simulink model "Milestone3_Code_JanasWork"  (R2023a)
settings: Solver=FixedStepDiscrete  StartTime=0.0  StopTime=100  FixedStep=0.01  RelTol=1e-3  EnableMultiTasking=on
undefined symbols (not defined in the file): DiscIntNeverNeededParam
libraries: arduinolib x14, simulink x3, hdlsllib x2, slpidlib x1, mobileRoboticsTrainingLib x1, arduinosensorlib x1
(part 1 of 2)
settings Model: NumberOfSteps=50  PacingRate=1000  ExtModeTrigDuration=2  Creator=Boitumelo  LastModifiedBy=27747
settings OptimizationCC: EnhancedBackFolding=on  PassReuseOutputArgsAs=Individual arguments  ZeroExternalMemoryAtStartup=off  ZeroInternalMemoryAtStartup=off  MaxStackSize=64  OptimizeBlockOrder=speed  DifferentSizesBufferReuse=on  OptimizationCustomize=off  EfficientTunableParamExpr=on
settings DebuggingCC: ParameterTunabilityLossMsg=error  UnconnectedInputMsg=warning  UnconnectedOutputMsg=warning  UnconnectedLineMsg=warning
settings HardwareCC: ProdBitPerPointer=32  ProdBitPerSizeT=32  ProdBitPerPtrDiffT=32  ProdLargestAtomicInteger=Long  ProdLargestAtomicFloat=Double  ProdWordSize=32  ProdHWDeviceType=ARM Compatible->ARM Cortex  UseEmbeddedCoderFeatures=off  UseSimulinkCoderFeatures=off
settings ModelReferenceCC: EnableRefExpFcnMdlSchedulingChecks=on
settings SFSimCC: MATLABDynamicMemAlloc=off
settings RTWCC: Description=Embedded Coder  SystemTargetFile=ert.tlc  HardwareBoard=Arduino Nano 33 IoT  TemplateMakefile=ert_default_tmf  Toolchain=Arduino ARM  BuildConfiguration=Faster Runs  DLArmComputeVersion=19.05
settings CodeAppCC: ForceParamTrailComments=on  IgnoreCustomStorageClasses=off  OperatorAnnotations=on  SimulinkDataObjDesc=on  SFDataObjDesc=on  InsertBlockDesc=on
settings ERTTargetCC: SupportContinuousTime=on  SupportNonInlinedSFcns=on  SupportVariableSizeSignals=on  ExtModeTransport=2  ExtModeStaticAlloc=on  ExtModeAutomaticAllocSize=off  ExtModeStaticAllocSize=8192  ExtModeMexFile=ext_xcp  ExtModeIntrfLevel=Level2 - Open

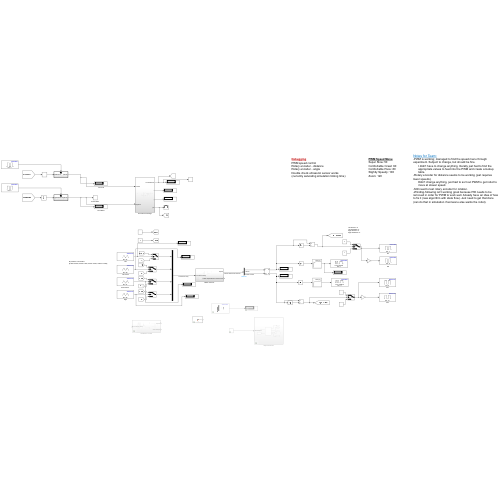
[thumbnail: Simulink's stored preview of the top-level diagram]
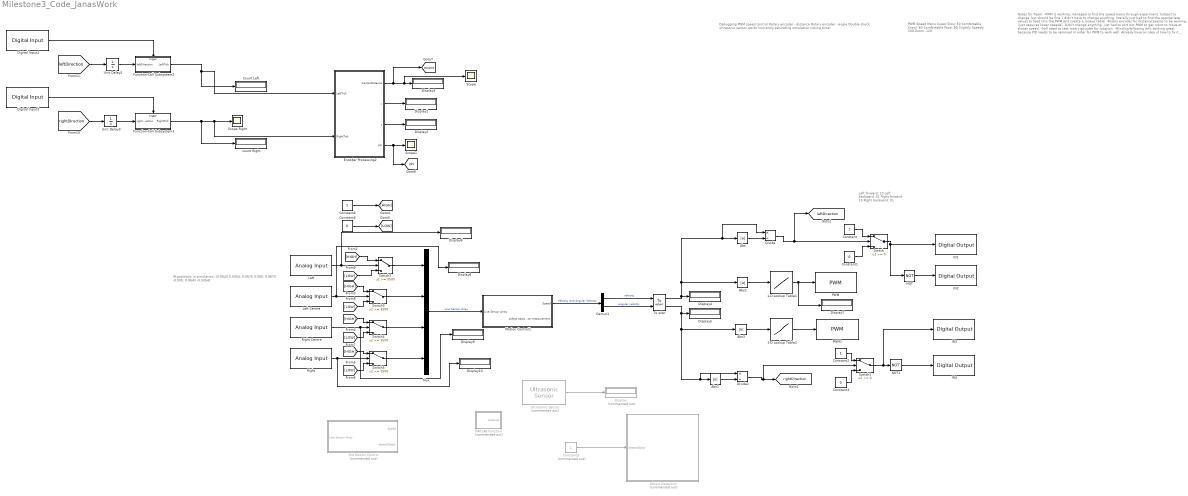
== system Milestone3_Code_JanasWork ==
  note: Notes for Team:
      | -PWM is working; managed to find the speed menu through experiment. Subject to change, but should be fine.
      | I didn't have to change anything, literally just had to find the appropriate values to feed into the PWM and create a lookup table.
      | -Rotary encoder for distance seems to be working (just requires lower speeds).
      | Didn't change anything, just had to sort out PWM to get robot to move at slower speed.
      | -Still need to test rotary encoder for rotation.
      | -Winding-following isn't working great because PID needs to be removed in order for PWM to work well. Already have an idea of how to fix it (new algorithm with state flow). Just need to get that done (can do that in simulation if someone else wants the robot).
  note: PWM Speed Menu
      | Super Slow: 50
      | Comfortable Crawl: 60
      | Comfortable Pace: 80
      | Slightly Speedy: 100
      | Zoom: 120
  note: Debugging
      | PWM speed control
      | Rotary encoder - distance
      | Rotary encoder - angle
      | Double check ultrasonic sensor works (currently saturating simulation ticking time)
  note: Left forward: 10
      | Left backward: 01
      | Right forward: 10
      | Right backward: 01
  note: IR positions in simulation:
      | [0.0643 0.0354; 0.0675 0.005; 0.0675 -0.005; 0.0643 -0.0354]
  1-D Lookup Table1 : Lookup_n-D  NumberOfTableDimensions=1  BreakpointsForDimension1=[0;1;2.19;30.06;32.26]  Table=[0;65;70;80;80]  InternalRulePriority=Speed  RndMeth=Simplest
  1-D Lookup Table2 : Lookup_n-D  NumberOfTableDimensions=1  BreakpointsForDimension1=[0;1;2.19;30.06;32.26]  Table=[0;65;70;80;92]  InternalRulePriority=Speed  RndMeth=Simplest
  Abs{,1..3} (4 alike) : Abs  SaturateOnIntegerOverflow=off
  Constant : Constant
  Constant1 : Constant  Value=0
  Constant2 : Constant
  Constant3 : Constant  Value=0
  Constant4 : Constant
  Constant5 : Constant  Commented=on
  Constant6 : Constant  Value=0
  Count Left : Display
  Demux1 : Demux  Outputs=2
  Digital Input2 : arduinolib/Digital Input  pinNumber=3  mode=Default  Direction=input  SampleTime=0.1  blockPlatform=arduino
  Digital Input3 : arduinolib/Digital Input  pinNumber=2  mode=Default  Direction=input  SampleTime=0.1  blockPlatform=arduino
  Display : Display  Commented=on
  Display{1..10} (10 alike) : Display
  Divide : Product  Inputs=*/
  Divide1 : Product  Inputs=*/
  Encoder Processing2 : Subsystem
  Function-Call Subsystem2 : Subsystem  TreatAsAtomicUnit=on
  Function-Call Subsystem3 : Subsystem  TreatAsAtomicUnit=on
  IN1 : arduinolib/Digital Output  pinNumber=7  Direction=output  blockPlatform=arduino
  IN2 : arduinolib/Digital Output  pinNumber=8  Direction=output  blockPlatform=arduino
  IN3 : arduinolib/Digital Output  pinNumber=9  Direction=output  blockPlatform=arduino
  IN4 : arduinolib/Digital Output  pinNumber=10  Direction=output  blockPlatform=arduino
  Left : arduinolib/Analog Input  pinNumber=7  ReadResultsOnly=off  ConversionTriggerSource=Software  ExternalTriggerType=uint32( 0 )  OutputDataType=uint16  EnableConversionCompleteNotify=off  EnableOuputStatus=off  SampleTime=-1  blockPlatform=arduino
  Left Centre : arduinolib/Analog Input  pinNumber=0  ReadResultsOnly=off  ConversionTriggerSource=Software  ExternalTriggerType=uint32( 0 )  OutputDataType=uint16  EnableConversionCompleteNotify=off  EnableOuputStatus=off  SampleTime=-1  blockPlatform=arduino
  MATLAB Function : MATLAB Function  Commented=on  TreatAsAtomicUnit=on
  Motion Control1 : Subsystem
  Mux : Mux
  NOT : Logic  Operator=NOT  IconShape=distinctive  AllPortsSameDT=off  OutDataTypeStr=boolean
  NOT1 : Logic  Operator=NOT  IconShape=distinctive  AllPortsSameDT=off  OutDataTypeStr=boolean
  Object Detection : Subsystem  Commented=on
  Old Motion Control : Subsystem  Commented=on
  PWM : arduinolib/PWM  pinNumber=6  frequencyType=Default  desiredFrequency=490.2  achievableFrequency=490.2
  PWM1 : arduinolib/PWM  pinNumber=11  frequencyType=Default  desiredFrequency=490.2  achievableFrequency=490.2
  Right : arduinolib/Analog Input  pinNumber=2  ReadResultsOnly=off  ConversionTriggerSource=Software  ExternalTriggerType=uint32( 0 )  OutputDataType=uint16  EnableConversionCompleteNotify=off  EnableOuputStatus=off  SampleTime=-1  blockPlatform=arduino
  Right Centre : arduinolib/Analog Input  pinNumber=1  ReadResultsOnly=off  ConversionTriggerSource=Software  ExternalTriggerType=uint32( 0 )  OutputDataType=uint16  EnableConversionCompleteNotify=off  EnableOuputStatus=off  SampleTime=-1  blockPlatform=arduino
  Scope : Scope
  Scope Right : Scope
  Scope1 : Scope
  Switch : Switch  SaturateOnIntegerOverflow=off  InputSameDT=off
  Switch1 : Switch  SaturateOnIntegerOverflow=off  InputSameDT=off
  Switch{2..5} (4 alike) : Switch  Threshold=3500  SaturateOnIntegerOverflow=off  InputSameDT=off
  To wlwr : mobileRoboticsTrainingLib/To wlwr  axleLength=0.17  wheelR=0.031
      link override change parameters: Gain=[1 -0.136/2; 1 0.136/2]
      link override vtow: Gain=1/0.031
  Ultrasonic Sensor : arduinosensorlib/Ultrasonic Sensor  Commented=on  NumSignalPins=1  TrigPin=4  EchoPin=5  SignalPin=3  SampleTime_=0.1  blockPlatform=ARDUINO
  Unit Delay2 : UnitDelay  SampleTime=-1  HasFrameUpgradeWarning=on
  Unit Delay3 : UnitDelay  SampleTime=-1  HasFrameUpgradeWarning=on
  count Right : Display
  tag scope: Distance=global, leftDirection=global, phi=global, rightDirection=global
  wires:
  Mux/1 -> Motion Control1/1(Line Sensor Array)  "Line Sensor Array"
  Abs/1 -> Divide/2
  Divide/1 -> [leftDirection], Switch/2
  Divide1/1 -> Switch1/2, [rightDirection]
  Abs1/1 -> Divide1/2
  To wlwr/2 -> Abs3/1, Divide1/1, Abs1/1, Display5/1
  Constant/1 -> Switch/1
  Switch/1 -> NOT/1, IN1/1
  Constant1/1 -> Switch/3
  NOT/1 -> IN2/1
  Constant2/1 -> Switch1/1
  Switch1/1 -> NOT1/1, IN3/1
  Constant3/1 -> Switch1/3
  NOT1/1 -> IN4/1
  Constant5/1 -> Object Detection/1(detectObject)
  [HIGH] -> Switch2/1
  [HIGH] -> Switch3/1
  [HIGH] -> Switch4/1
  [HIGH] -> Switch5/1
  [LOW] -> Switch5/3
  [LOW] -> Switch4/3
  [LOW] -> Switch3/3
  [LOW] -> Switch2/3
  Left/1 -> Display6/1, Switch2/2
  Right Centre/1 -> Display9/1, Switch4/2
  Right/1 -> Switch5/2, Display10/1
  Switch2/1 -> Mux/1
  Switch3/1 -> Mux/2
  Switch4/1 -> Mux/3
  Switch5/1 -> Mux/4
  Constant4/1 -> [HIGH]
  Constant6/1 -> [LOW]
  Abs2/1 -> 1-D Lookup Table1/1
  1-D Lookup Table1/1 -> PWM/1, Display7/1
  Abs3/1 -> 1-D Lookup Table2/1
  1-D Lookup Table2/1 -> PWM1/1
  Ultrasonic Sensor/1 -> Display/1
  [rightDirection] -> Unit Delay3/1
  Unit Delay3/1 -> Function-Call Subsystem3/1(rightDirection)
  Unit Delay2/1 -> Function-Call Subsystem2/1(leftDirection)
  Encoder Processing2/3(y) -> Display2/1
  Encoder Processing2/2(x) -> Display1/1
  Digital Input3/1 -> Function-Call Subsystem3/Trigger
  Encoder Processing2/1(CenterDistance) -> Scope/1, Display3/1, [Distance]
  Digital Input2/1 -> Function-Call Subsystem2/Trigger
  [leftDirection] -> Unit Delay2/1
  Function-Call Subsystem2/1(LeftTick) -> Count Left/1, Encoder Processing2/1(LeftTick)
  Encoder Processing2/4(phi) -> [phi], Scope1/1
  Function-Call Subsystem3/1(RightTick) -> count Right/1, Encoder Processing2/2(RightTick), Scope Right/1
  Left Centre/1 -> Switch3/2, Display8/1
  Motion Control1/1(Speed) -> Demux1/1  "Velocity and Angular Velocity"
  To wlwr/1 -> Abs2/1, Divide/1, Abs/1, Display4/1
  Demux1/1 -> To wlwr/1  "velocity"
  Demux1/2 -> To wlwr/2  "angular velocity"

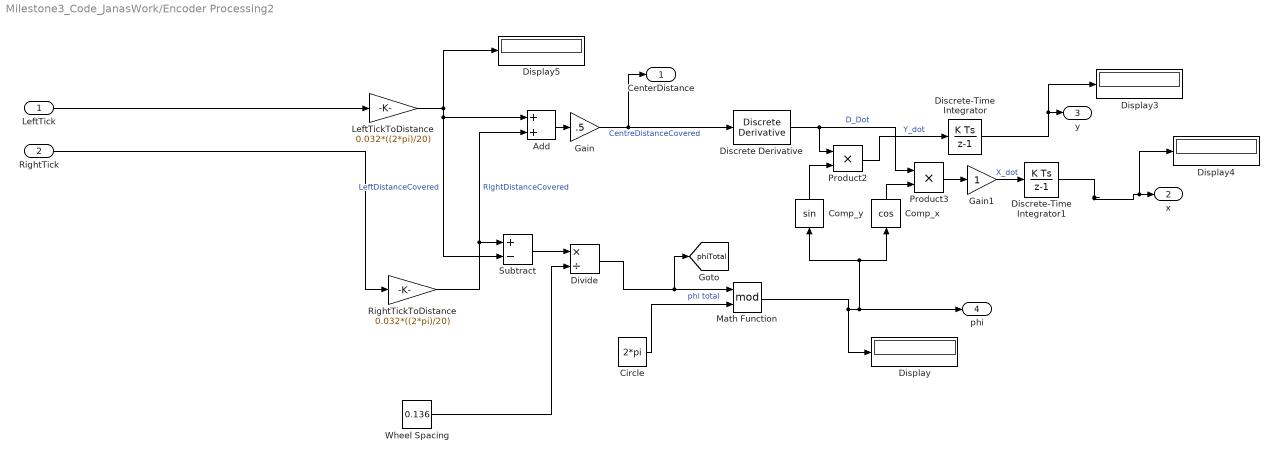
== system Milestone3_Code_JanasWork/Encoder Processing2 ==
  LeftTick : Inport
  RightTick : Inport  Port=2
  Add : Sum
  Circle : Constant  Value=2*pi
  Comp_x : Trigonometry  Operator=cos
  Comp_y : Trigonometry
  Discrete Derivative : simulink/Discrete/Discrete Derivative  gainval=1.0  ICPrevScaledInput=0.0  OutMin=[]  OutMax=[]  OutDataType=fixdt(1, 16)  OutScaling=2^-10  DoSatur=off
  Discrete-Time Integrator : DiscreteIntegrator  SampleTime=-1  ICPrevOutput=DiscIntNeverNeededParam  ICPrevScaledInput=DiscIntNeverNeededParam
  Discrete-Time Integrator1 : DiscreteIntegrator  SampleTime=-1  ICPrevOutput=DiscIntNeverNeededParam  ICPrevScaledInput=DiscIntNeverNeededParam
  Display{,3..5} (4 alike) : Display
  Divide : Product  Inputs=*/
  Gain : Gain  Gain=.5
  Gain1 : Gain
  LeftTickToDistance : Gain  Gain=0.032*((2*pi)/20)
  Math Function : Math  Operator=mod  SignedPower=on
  Product2 : Product
  Product3 : Product
  RightTickToDistance : Gain  Gain=0.032*((2*pi)/20)
  Subtract : Sum  Inputs=+-
  Wheel Spacing : Constant  Value=0.136
  CenterDistance : Outport
  x : Outport  Port=2
  y : Outport  Port=3
  phi : Outport  Port=4
  tag scope: phiTotal=global
  wires:
  Divide/1 -> [phiTotal], Math Function/1  "phi total"
  Gain/1 -> Discrete Derivative/1, CenterDistance/1  "CentreDistanceCovered"
  Subtract/1 -> Divide/1
  Add/1 -> Gain/1
  RightTickToDistance/1 -> Subtract/1, Add/2  "RightDistanceCovered"
  RightTick/1 -> RightTickToDistance/1
  LeftTickToDistance/1 -> Add/1, Subtract/2, Display5/1  "LeftDistanceCovered"
  Comp_y/1 -> Product2/2
  Comp_x/1 -> Product3/2
  LeftTick/1 -> LeftTickToDistance/1
  Product2/1 -> Discrete-Time Integrator/1  "Y_dot"
  Product3/1 -> Gain1/1
  Wheel Spacing/1 -> Divide/2
  Circle/1 -> Math Function/2
  Discrete Derivative/1 -> Product3/1, Product2/1  "D_Dot"
  Gain1/1 -> Discrete-Time Integrator1/1  "X_dot"
  Math Function/1 -> Comp_x/1, Comp_y/1, phi/1, Display/1
  Discrete-Time Integrator1/1 -> Display4/1, x/1
  Discrete-Time Integrator/1 -> Display3/1, y/1

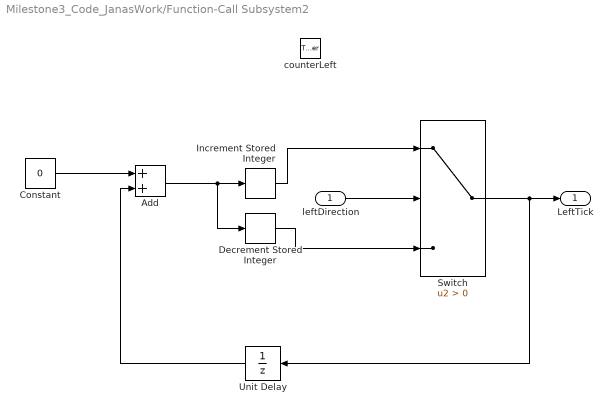
== system Milestone3_Code_JanasWork/Function-Call Subsystem2 ==
  leftDirection : Inport
  counterLeft : TriggerPort  TriggerType=either  FunctionName=counterLeft  VariantControl=(inherit)
  Add : Sum
  Constant : Constant  Value=0
  Decrement Stored Integer : simulink/Additional Math & Discrete/Additional Math: Increment - Decrement/Decrement Stored Integer
  Increment Stored Integer : hdlsllib/Math Operations/Increment Stored Integer
  Switch : Switch  Criteria=u2 > Threshold  SaturateOnIntegerOverflow=off  InputSameDT=off
  Unit Delay : UnitDelay  SampleTime=-1  HasFrameUpgradeWarning=on
  LeftTick : Outport
  wires:
  Decrement Stored Integer/1 -> Switch/3
  Increment Stored Integer/1 -> Switch/1
  Unit Delay/1 -> Add/2
  leftDirection/1 -> Switch/2
  Constant/1 -> Add/1
  Switch/1 -> Unit Delay/1, LeftTick/1
  Add/1 -> Decrement Stored Integer/1, Increment Stored Integer/1

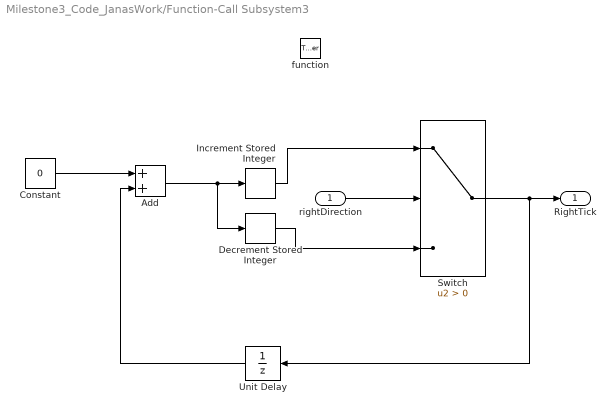
== system Milestone3_Code_JanasWork/Function-Call Subsystem3 ==
  rightDirection : Inport
  function : TriggerPort  TriggerType=either  VariantControl=(inherit)
  Add : Sum
  Constant : Constant  Value=0
  Decrement Stored Integer : simulink/Additional Math & Discrete/Additional Math: Increment - Decrement/Decrement Stored Integer
  Increment Stored Integer : hdlsllib/Math Operations/Increment Stored Integer
  Switch : Switch  Criteria=u2 > Threshold  SaturateOnIntegerOverflow=off  InputSameDT=off
  Unit Delay : UnitDelay  SampleTime=-1  HasFrameUpgradeWarning=on
  RightTick : Outport
  wires:
  Decrement Stored Integer/1 -> Switch/3
  Increment Stored Integer/1 -> Switch/1
  Unit Delay/1 -> Add/2
  rightDirection/1 -> Switch/2
  Constant/1 -> Add/1
  Switch/1 -> Unit Delay/1, RightTick/1
  Add/1 -> Decrement Stored Integer/1, Increment Stored Integer/1

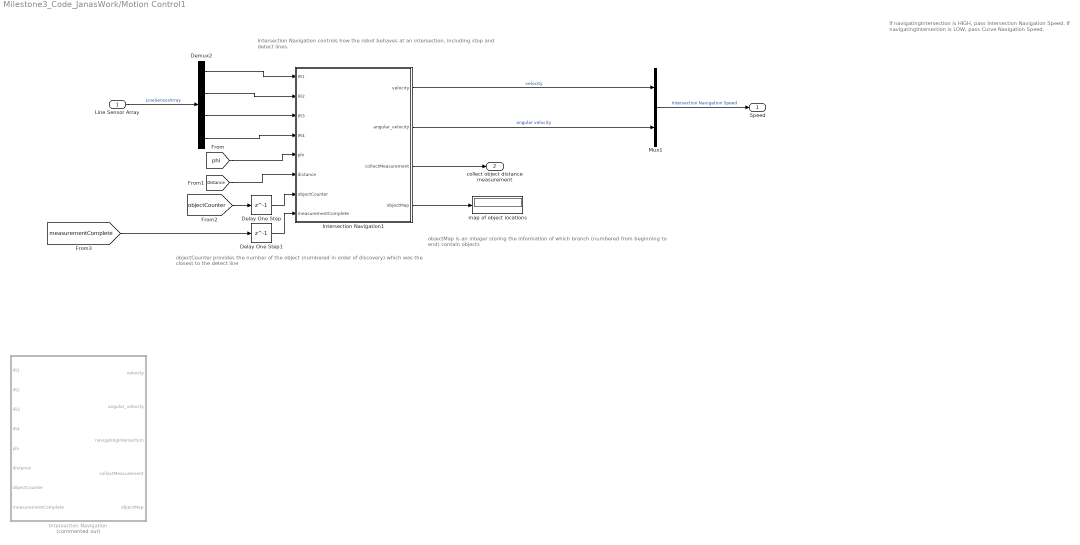
== system Milestone3_Code_JanasWork/Motion Control1 ==
  note: objectCounter provides the number of the object (numbered in order of discovery) which was the closest to the detect line
  note: objectMap is an integer storing the information of which branch (numbered from beginning to end) contain objects
  note: Intersection Navigation controls how the robot behaves at an intersection, including stop and detect lines.
  note: If navigatingIntersection is HIGH, pass Intersection Navigation Speed.
      | If navigatingIntersection is LOW, pass Curve Navigation Speed.
  Line Sensor Array : Inport
  Delay One Step : Delay  DelayLength=1
  Delay One Step1 : Delay  DelayLength=1
  Demux2 : Demux
  Intersection Navigation : Stateflow chart  Commented=on  TreatAsAtomicUnit=on
  Intersection Navigation1 : Stateflow chart  TreatAsAtomicUnit=on
  Mux1 : Mux  Inputs=2
  map of object locations : Display
  Speed : Outport
  collect object distance measurement : Outport  Port=2
  wires:
  Intersection Navigation1/3(collectMeasurement) -> collect object distance measurement/1
  Demux2/1 -> Intersection Navigation1/1(IR1)
  Demux2/3 -> Intersection Navigation1/3(IR3)
  Demux2/2 -> Intersection Navigation1/2(IR2)
  Demux2/4 -> Intersection Navigation1/4(IR4)
  Intersection Navigation1/1(velocity) -> Mux1/1  "velocity"
  Intersection Navigation1/2(angular_velocity) -> Mux1/2  "angular velocity"
  Line Sensor Array/1 -> Demux2/1  "LineSensorArray"
  [phi] -> Intersection Navigation1/5(phi)
  [Distance] -> Intersection Navigation1/6(distance)
  Intersection Navigation1/4(objectMap) -> map of object locations/1
  [objectCounter] -> Delay One Step/1
  Delay One Step/1 -> Intersection Navigation1/7(objectCounter)
  [measurementComplete] -> Delay One Step1/1
  Delay One Step1/1 -> Intersection Navigation1/8(measurementComplete)
  Mux1/1 -> Speed/1  "Intersection Navigation Speed"

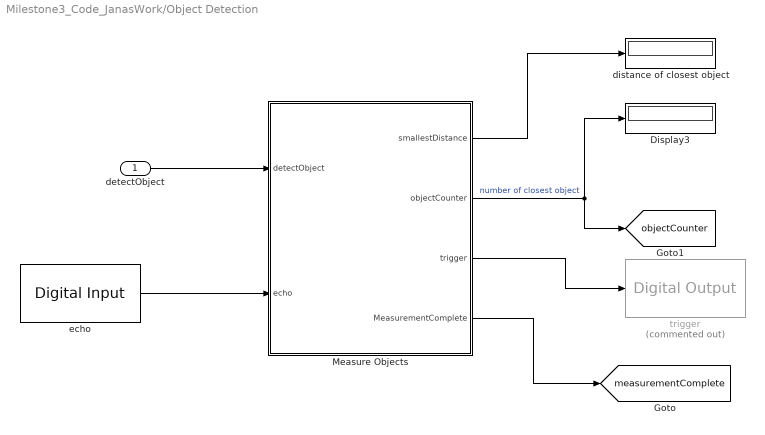
== system Milestone3_Code_JanasWork/Object Detection ==
  detectObject : Inport
  Display3 : Display
  Measure Objects : Stateflow chart  TreatAsAtomicUnit=on
  distance of closest object : Display
  echo : arduinolib/Digital Input  pinNumber=0  mode=Default  Direction=input  SampleTime=0.1  blockPlatform=arduino
  trigger : arduinolib/Digital Output  Commented=on  pinNumber=1  Direction=output  blockPlatform=arduino
  tag scope: measurementComplete=global, objectCounter=global
  wires:
  detectObject/1 -> Measure Objects/1(detectObject)
  Measure Objects/1(smallestDistance) -> distance of closest object/1
  Measure Objects/2(objectCounter) -> [objectCounter], Display3/1  "number of closest object"
  Measure Objects/3(trigger) -> trigger/1
  echo/1 -> Measure Objects/2(echo)
  Measure Objects/4(MeasurementComplete) -> [measurementComplete]

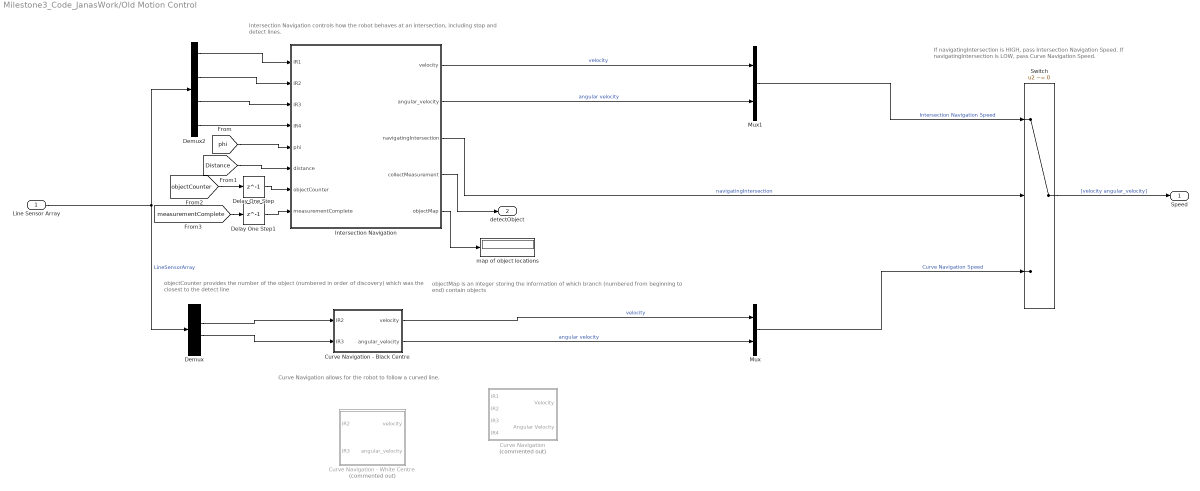
== system Milestone3_Code_JanasWork/Old Motion Control ==
  note: objectCounter provides the number of the object (numbered in order of discovery) which was the closest to the detect line
  note: objectMap is an integer storing the information of which branch (numbered from beginning to end) contain objects
  note: Intersection Navigation controls how the robot behaves at an intersection, including stop and detect lines.
  note: Curve Navigation allows for the robot to follow a curved line.
  note: If navigatingIntersection is HIGH, pass Intersection Navigation Speed.
      | If navigatingIntersection is LOW, pass Curve Navigation Speed.
  Line Sensor Array : Inport
  Curve Navigation : Subsystem  Commented=on
  Curve Navigation - Black Centre : Stateflow chart  TreatAsAtomicUnit=on
  Curve Navigation - White Centre : Stateflow chart  Commented=on  TreatAsAtomicUnit=on
  Delay One Step : Delay  DelayLength=1
  Delay One Step1 : Delay  DelayLength=1
  Demux : Demux
  Demux2 : Demux
  Intersection Navigation : Stateflow chart  TreatAsAtomicUnit=on
  Mux : Mux  Inputs=2
  Mux1 : Mux  Inputs=2
  Switch : Switch  Criteria=u2 ~= 0  Threshold=1  SaturateOnIntegerOverflow=off  InputSameDT=off
  map of object locations : Display
  Speed : Outport
  detectObject : Outport  Port=2
  wires:
  Intersection Navigation/4(collectMeasurement) -> detectObject/1
  Curve Navigation - Black Centre/1(velocity) -> Mux/1  "velocity"
  Mux1/1 -> Switch/1  "Intersection Navigation Speed"
  Intersection Navigation/3(navigatingIntersection) -> Switch/2  "navigatingIntersection"
  Demux2/1 -> Intersection Navigation/1(IR1)
  Demux2/3 -> Intersection Navigation/3(IR3)
  Demux2/2 -> Intersection Navigation/2(IR2)
  Demux2/4 -> Intersection Navigation/4(IR4)
  Intersection Navigation/1(velocity) -> Mux1/1  "velocity"
  Intersection Navigation/2(angular_velocity) -> Mux1/2  "angular velocity"
  Mux/1 -> Switch/3  "Curve Navigation Speed"
  Switch/1 -> Speed/1  "[velocity angular_velocity]"
  Curve Navigation - Black Centre/2(angular_velocity) -> Mux/2  "angular velocity"
  Demux/2 -> Curve Navigation - Black Centre/1(IR2)
  Demux/3 -> Curve Navigation - Black Centre/2(IR3)
  Line Sensor Array/1 -> Demux/1, Demux2/1  "LineSensorArray"
  [phi] -> Intersection Navigation/5(phi)
  [Distance] -> Intersection Navigation/6(distance)
  Intersection Navigation/5(objectMap) -> map of object locations/1
  [objectCounter] -> Delay One Step/1
  Delay One Step/1 -> Intersection Navigation/7(objectCounter)
  Delay One Step1/1 -> Intersection Navigation/8(measurementComplete)
  [measurementComplete] -> Delay One Step1/1

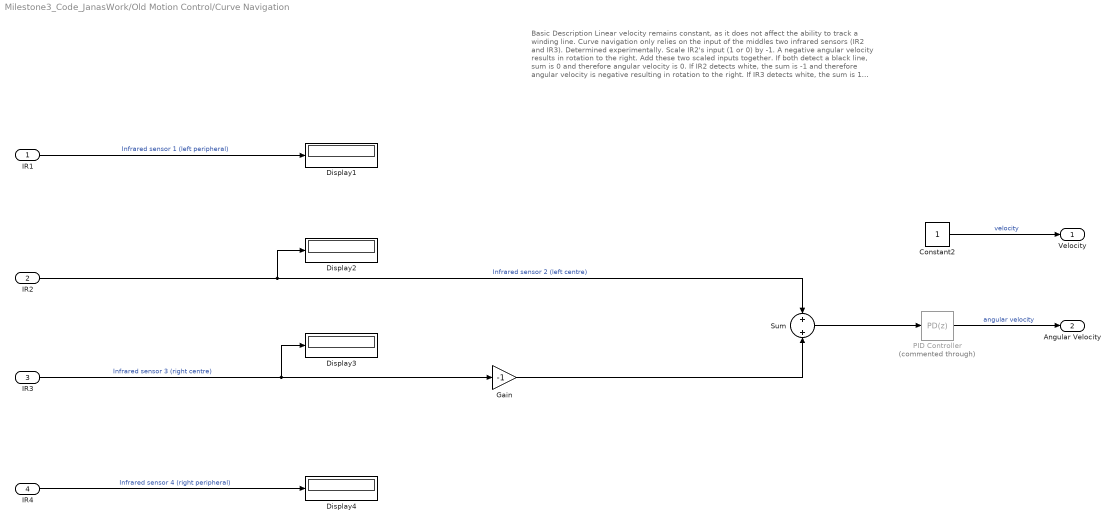
== system Milestone3_Code_JanasWork/Old Motion Control/Curve Navigation ==
  note: Basic Description
      | Linear velocity remains constant, as it does not affect the ability to track a winding line.
      | Curve navigation only relies on the input of the middles two infrared sensors (IR2 and IR3).
      | Determined experimentally.
      | Scale IR2's input (1 or 0) by -1.
      | A negative angular velocity results in rotation to the right.
      | Add these two scaled inputs together.
      | If both detect a black line, sum is 0 and therefore angular velocity is 0.
      | If IR2 detects white, the sum is -1 and therefore angular velocity is negative resulting
      | in rotation to the right.
      | If IR3 detects white, the sum is 1 and therefore the angular velocity is positive r
      | esulting in rotation to the left.
      | Pass inputs to a PID to scale appropriately.
      | Set angular velocity to the output of the PID.
  IR1 : Inport
  IR2 : Inport  Port=2
  IR3 : Inport  Port=3
  IR4 : Inport  Port=4
  Constant2 : Constant
  Display{1..4} (4 alike) : Display
  Gain : Gain  Gain=-1
  PID Controller : slpidlib/PID Controller  Commented=through  Controller=PD  Form=Parallel  TimeDomain=Discrete-time  UseExternalTs=off  SampleTime=-1  IntegratorMethod=Forward Euler  FilterMethod=Forward Euler  ControllerParametersSource=internal  P=25  I=0  UseKiTs=off  D=1  N=100  UseFilter=on  TunerSelectOption=Transfer Function Based (PID Tuner App)  InitialConditionSource=internal  InitialConditionForIntegrator=0  InitialConditionForFilter=0  DifferentiatorICPrevScaledInput=0  ExternalReset=none  TrackingMode=off  Kt=1  LimitOutput=off  SatLimitsSource=internal  UpperSaturationLimit=inf  LowerSaturationLimit=-inf  LinearizeAsGain=on  AntiWindupMode=none  Kb=1  LimitIntegrator=off  UpperIntegratorSaturationLimit=inf  LowerIntegratorSaturationLimit=-inf  PGainOutDataTypeStr=double  PProdOutDataTypeStr=double  POutMin=[]  POutMax=[]  IOutMin=[]  IOutMax=[]  DGainOutDataTypeStr=double  DProdOutDataTypeStr=double  DOutMin=[]  DOutMax=[]  NGainOutDataTypeStr=double  NProdOutDataTypeStr=double  NOutMin=[]  NOutMax=[]  SumOutDataTypeStr=double  SumOutMin=[]  SumOutMax=[]  SaturationOutMin=[]  SaturationOutMax=[]  PParamMin=[]  PParamMax=[]  IParamMin=[]  IParamMax=[]  DParamMin=[]  DParamMax=[]  NParamMin=[]  NParamMax=[]  KbParamMin=[]  KbParamMax=[]  KtParamMin=[]  KtParamMax=[]  KbOutMin=[]  KbOutMax=[]  KtOutMin=[]  KtOutMax=[]  IntegratorOutMin=[]  IntegratorOutMax=[]  FilterOutMin=[]  FilterOutMax=[]  SumI1OutMin=[]  SumI1OutMax=[]  SumI2OutMin=[]  SumI2OutMax=[]  SumI3OutMin=[]  SumI3OutMax=[]  SumI4OutMin=[]  SumI4OutMax=[]  SumDOutMin=[]  SumDOutMax=[]  DifferentiatorOutMin=[]  DifferentiatorOutMax=[]  FilterDiffOutCoefMin=[]  FilterDiffOutCoefMax=[]  ReciprocalOutMin=[]  ReciprocalOutMax=[]  SumDenOutMin=[]  SumDenOutMax=[]  SumNumOutMin=[]  SumNumOutMax=[]  DivideOutMin=[]  DivideOutMax=[]  UdiffTsProdOutMin=[]  UdiffTsProdOutMax=[]  NTsProdOutMin=[]  NTsProdOutMax=[]  UintegralTsProdOutMin=[]  UintegralTsProdOutMax=[]  UngainTsProdOutMin=[]  UngainTsProdOutMax=[]  ClampingZeroOutDataTypeStr=Inherit: Inherit via back propagation  ClampingZeroOutMin=[]  ClampingZeroOutMax=[]  FilterDenConstantOutDataTypeStr=Inherit: Inherit via back propagation  FilterDenConstantOutMin=[]  FilterDenConstantOutMax=[]  PCopyOutDataTypeStr=Inherit: Inherit via back propagation  PCopyOutMin=[]  PCopyOutMax=[]  NCopyOutDataTypeStr=Inherit: Inherit via back propagation  NCopyOutMin=[]  NCopyOutMax=[]  IntegratorContinuousStateAttributes=''  IntegratorStateMustResolveToSignalObject=off  IntegratorRTWStateStorageClass=Auto  FilterContinuousStateAttributes=''  FilterStateMustResolveToSignalObject=off  FilterRTWStateStorageClass=Auto  ParallelPVariant=InternalParameters  IdealPVariant=Disabled  IVariant=Disabled  DVariant=InternalParameters  IntegratorVariant=Disabled  SatVariant=Disabled  AWVariant=Disabled  PCopyVariant=Disabled  TRVariant=Disabled  FdbkBlocksVariant=Forward  IdealPFdbkVariant=Disabled  SatFdbkVariant=Disabled  DerivativeFilterVariant=ForwardEulerFilter  NVariant=InternalParameters  NCopyVariant=Disabled  FilterICVariant=InternalICsFilter  IntegratorICVariant=Disabled  ExternalResetVariant=Disabled  TRSumVariant=Passthrough  SumFdbkVariant=Disabled  SumVariant=Sum_PD  TsampFilterVariant=InternalTs  TsampNgainVariant=Passthrough  TsampIntegralVariant=Disabled_SignalSpec  ExternalSaturationOutDataTypeStr=Inherit: Same as second input
  Sum : Sum
  Velocity : Outport
  Angular Velocity : Outport  Port=2
  wires:
  IR1/1 -> Display1/1  "Infrared sensor 1 (left peripheral)"
  IR2/1 -> Sum/1, Display2/1  "Infrared sensor 2 (left centre)"
  IR3/1 -> Gain/1, Display3/1  "Infrared sensor 3 (right centre)"
  IR4/1 -> Display4/1  "Infrared sensor 4 (right peripheral)"
  Constant2/1 -> Velocity/1  "velocity"
  Sum/1 -> PID Controller/1
  PID Controller/1 -> Angular Velocity/1  "angular velocity"
  Gain/1 -> Sum/2

== stateflow chart Milestone3_Code_JanasWork/Old Motion Control/Intersection Navigation ==
  note: Basic Description
      | Default: Curve Navigation controls the velocity and angular velocity
      |
      | When infrared sensor 1 or 4 (IR1 and IR4) detect a black line, this Intersection Navigation subsystem takes control and calls the leftTurn or rightTurn procedure respectively.
      | Intersection procedure (same for both leftTurn or rightTurn):
      | 	Increment branchCounter to keep track of the number of branches.
      | 	Move forward a small distance to align with the turn.
      | 	Rotate in the correct direction until the middle two sensors detect a line again.
      | 	Pass control to Curve Navigation to navigate the offshoot.
      | 	If the offshoot comes to an end (all sensors detect white), rotate 180 degrees and navigate back to the main path.
      | 	If the offshoot ends in a detect line (all sensors detect black), stop, send a signal to the Object Detection subsystem to measure for an object, rotate 180 degrees and navigate back to the main path.
      | 		Add branch number from branchCounter to objectMap to indicate this branch has an object.
      | 	Pass control to Curve Navigation to navigate the offshoot returning to the main path.
      | 	When the peripheral sensors detect a black line again (meaning the robot has returned to the intersection with the main branch), control is passed to Intersection Navigation.
      | 	Move forward a small distance to align with the turn.
      | 	Rotate in the correct direction until the middle two sensors detect a line again.
      | 	Pass control back to Curve Navigation to continue traversing the main path.
      |
      | If all sensors detect black whilst the robot is on the main path, the endOfMaze procedure is called.
      | endOfMaze procedure:
      | 	Stop
      | 	Use objectMap to determine how many objects were discovered.
      | 	Find the branch number of the object with the smallest distance, saved to branchWithObject.
      | 		objectCounter provides number of object with smallest distance measured.
      | 		Obtain the n'th number in objectMap to determine the branch number containing said object (where n = objectCounter)
      | 	Invert branchWithObject such that it provides the number of the branch starting from the end of the maze.
      | 	Set renavigating to HIGH.
      |
      | Renavigating Procedure:
      | 	Rotate 180 degrees to re-traverse the maze.
      | 	set branchCounter to 0.
      | 	Pass control to Curve Navigation to renavigate maze.
      | 	If intersection is detected, increment branchCounter.
      | 	If branchCounter is equal to branchWithObject at an intersection, turn into that offshoot.
      | 	Pass control to Curve Navigation to navigate offshoot.
      | 	If all sensors detect black at the "detect object line", come to a stop.
  state endOfMaze
    %procedure to locate position of closest object once maze is completed
    entry: navigatingIntersection = 1;
    velocity = 0;
    angular_velocity = 0;
    num = objectMap;
    while num > 0
    len = len + 1;
    num = fix(num/10);
    end
    branchWithObject = mod(fix(objectMap/10^(len - objectCounter)), 10);
    branchWithObject = branchCounter - branchWithObject + 1;
    exit:
    renavigating = 1;
  state fullRotation
    %rotate 180 degrees to renavigate maze
    entry: phi0 = phi;
    during:
    velocity = 0;
    angular_velocity = -4;
  state mainPath
    %Control given to Curve Navigation Subsystem
    entry: navigatingIntersection = 0;
  state rightTurn
    %procedure for navigating an offshoot to the right of the main path
    state returnToMain
      entry: navigatingIntersection = 0;
    state rightToMain
      %turn right back onto the main path
      entry: phi0 = phi;
      during:
      velocity = 0.1;
      angular_velocity = -4;
    state alignWithTurn
      entry: distance0 = distance;
      branchCounter = branchCounter +1;
      exit: navigatingIntersection = 1;
    state alignWithMain
      entry: distance0 = distance;
      exit: navigatingIntersection = 1;
    state rotate
      %turn right
      entry:
      phi0 = phi;
      during:
      velocity = 0.1;
      angular_velocity = -4;
    state navigateOffshoot
      entry: navigatingIntersection = 0;
      exit: navigatingIntersection = 1;
    state stopAndMeasure
      entry:
      velocity = 0;
      angular_velocity = 0;
      collectMeasurement = 1;
      exit:
      collectMeasurement = 0;
    state fullRotation
      %rotate 180 degrees
      entry: phi0 = phi;
      during:
      velocity = 0;
      angular_velocity = -4;
    state finalStop
      velocity = 0;
      angular_velocity = 0;
    (default) -> rightTurn.alignWithTurn
    rightTurn.alignWithMain -> rightToMain : [abs(distance - distance0) > 0.01]
    rightTurn.returnToMain -> rightTurn.alignWithMain : [IR4 == 0]
    rightTurn.alignWithTurn -> rightTurn.rotate : [abs(distance - distance0) > 0.005]
    rightTurn.fullRotation -> rightTurn.returnToMain : [abs(phi - phi0) > 2.793 && abs(phi - phi0) < 3.491 && IR2 == 0 && IR3 == 0]
    rightTurn.rotate -> rightTurn.navigateOffshoot : [((abs(phi - phi0) > 0.3491 && abs(phi - phi0) < 2.967) || (abs(phi - phi0) > 3.316 && abs(phi - phi0) < 5.934)) && IR2 == 0 && IR3 == 0]
    rightTurn.navigateOffshoot -> (junction 254) [order 1]
    rightTurn.navigateOffshoot -> (junction 194) [order 3] : [IR1 == 1 && IR2 == 1 && IR3 == 1 && IR4 == 1]
    (junction 254) -> (junction 256) : [IR1 + IR2 + IR3 + IR4 == 0 && renavigating == 1]
    (junction 194) -> rightTurn.fullRotation
    rightTurn.navigateOffshoot -> rightTurn.stopAndMeasure [order 2] : [IR1 == 0 && IR2 == 0 && IR3 == 0 && IR4 ==0]{objectMap = objectMap*10 + branchCounter;} %detect or stop line
    rightTurn.stopAndMeasure -> rightTurn.fullRotation : [measurementComplete == 1]
    (junction 256) -> rightTurn.finalStop
  state leftTurn
    %procedure for navigating an offshoot to the right of the main path
    state leftToMain
      %turn left back onto the main path
      entry: phi0 = phi;
      during:
      velocity = 0.1;
      angular_velocity = 4;
    state returnToMain
      entry: navigatingIntersection = 0;
    state alignWithTurn
      entry: distance0 = distance;
      branchCounter = branchCounter +1;
      exit: navigatingIntersection = 1;
    state alignWithMain
      entry: distance0 = distance;
      exit: navigatingIntersection = 1;
    state rotate
      %turn left
      entry:
      phi0 = phi;
      during:
      velocity = 0.1;
      angular_velocity = 4;
    state navigateOffshoot
      entry: navigatingIntersection = 0;
      exit: navigatingIntersection = 1;
    state stopAndMeasure
      entry:
      velocity = 0;
      angular_velocity = 0;
      collectMeasurement = 1;
      exit:
      collectMeasurement = 0;
    state fullRotation
      %rotate 180 degrees
      entry: phi0 = phi;
      during:
      velocity = 0;
      angular_velocity = -4;
    state finalStop
      velocity = 0;
      angular_velocity = 0;
    (default) -> leftTurn.alignWithTurn
    leftTurn.alignWithMain -> leftToMain : [abs(distance - distance0) > 0.01]
    leftTurn.returnToMain -> leftTurn.alignWithMain : [IR1 == 0]
    leftTurn.alignWithTurn -> leftTurn.rotate : [abs(distance - distance0) > 0.005]
    leftTurn.fullRotation -> leftTurn.returnToMain : [abs(phi - phi0) > 2.793 && abs(phi - phi0) < 3.491 && IR2 == 0 && IR3 == 0]
    leftTurn.rotate -> leftTurn.navigateOffshoot : [((abs(phi - phi0) > 0.3491 && abs(phi - phi0) < 2.967) || (abs(phi - phi0) > 3.316 && abs(phi - phi0) < 5.934)) && IR2 == 0 && IR3 == 0]
    leftTurn.navigateOffshoot -> (junction 216) [order 3] : [IR1 == 1 && IR2 == 1 && IR3 == 1 && IR4 == 1]
    leftTurn.navigateOffshoot -> (junction 263) [order 1]
    (junction 216) -> leftTurn.fullRotation
    (junction 263) -> (junction 264) : [IR1 + IR2 + IR3 + IR4 == 0 && renavigating == 1]
    leftTurn.navigateOffshoot -> leftTurn.stopAndMeasure [order 2] : [IR1 == 0 && IR2 == 0 && IR3 == 0 && IR4 ==0]{objectMap = objectMap*10 + branchCounter;} %detect or stop line
    leftTurn.stopAndMeasure -> leftTurn.fullRotation : [measurementComplete == 1]
    (junction 264) -> leftTurn.finalStop
  state renavigatingCounter
    entry:
    branchCounter = branchCounter + 1;
  endOfMaze -> fullRotation [commented out] : {branchCounter = 0;}
  fullRotation -> mainPath : [abs(phi - phi0) > 2.793 && abs(phi - phi0) < 3.491 && IR2 == 0 && IR3 == 0]
  mainPath -> endOfMaze [order 1] : [IR1 + IR2 + IR3 + IR4 == 0]
  (default) -> mainPath
  (junction 225) -> mainPath
  (junction 197) -> mainPath
  leftToMain -> (junction 225) : [((abs(phi - phi0) > 0.3491 && abs(phi - phi0) < 2.967) || (abs(phi - phi0) > 3.316 && abs(phi - phi0) < 5.934)) && IR2 == 0 && IR3 == 0]
  rightToMain -> (junction 197) : [((abs(phi - phi0) > 0.3491 && abs(phi - phi0) < 2.967) || (abs(phi - phi0) > 3.316 && abs(phi - phi0) < 5.934)) && IR2 == 0 && IR3 == 0]
  mainPath -> (junction 223) [order 3] : [IR1 == 0 && IR2 == 0 && IR3 == 0 && IR4 == 1 && ((renavigating == 0) || (renavigating == 1 && branchCounter == branchWithObject) )]
  renavigatingCounter -> mainPath [order 3] : [IR1 == 1 && IR4 == 1]
  mainPath -> renavigatingCounter [order 4] : [(IR1 == 0 || IR4 == 0) && renavigating == 1]
  mainPath -> (junction 199) [order 2] : [IR1 == 1 && IR2 == 0 && IR3 == 0 && IR4 == 0 && ((renavigating == 0) || (renavigating == 1 && branchCounter == branchWithObject) )]
  (junction 223) -> leftTurn
  (junction 199) -> rightTurn
  renavigatingCounter -> rightTurn.rotate [order 1] : [IR4 == 0 && branchCounter == branchWithObject]{navigatingIntersection = 1;}
  renavigatingCounter -> leftTurn.rotate [order 2] : [IR1 == 0 && branchCounter == branchWithObject]{navigatingIntersection = 1;}
  data: len local =0; num local =0; velocity output; angular_velocity output; IR1 input; IR2 input; IR3 input; IR4 input; navigatingIntersection output; collectMeasurement output; phi input; phi0 local; distance input; distance0 local =0; objectCounter input; objectMap output =0; branchCounter local =0; branchWithObject local =0; renavigating local =0; measurementComplete input

== matlab function Milestone3_Code_JanasWork/MATLAB Function ==
  data: distance output
function distance = fcn()
    %function called when trigger set high
    %arduinoObj = arduino('COM5', 'Nano 33 IOT', "Libraries", "Ultrasonic");
        arduinoObj = arduino('COM5', 'Nano33IoT', 'Libraries', 'Ultrasonic');

        ultrasonicObj = ultrasonic(arduinoObj,'D1','D0')
distance = readDistance(ultrasonicObj);

== stateflow chart Milestone3_Code_JanasWork/Old Motion Control/Curve Navigation - Black Centre ==
  state TurnRight
    entry:
    velocity = 0
    angular_velocity = 2
  state FollowTrack
    %middle two sense black
    velocity = 1
    angular_velocity = 0
  state TurnLeft
    entry:
    velocity = 0
    angular_velocity = -2
  (default) -> FollowTrack
  FollowTrack -> TurnLeft [order 1] : [IR3 == 1]
  TurnRight -> FollowTrack : [IR3 == 0 && IR2 == 0]
  TurnLeft -> FollowTrack : [IR3 == 0 && IR2 == 0]
  FollowTrack -> TurnRight [order 2] : [IR2 == 1]
  data: velocity output; angular_velocity output; IR2 input; IR3 input

== stateflow chart Milestone3_Code_JanasWork/Old Motion Control/Curve Navigation - White Centre ==
  state TurnRight
    entry:
    velocity = 0
    angular_velocity = 2
  state FollowTrack
    %middle two sense white
    velocity = 1
    angular_velocity = 0
  state TurnLeft
    entry:
    velocity = 0
    angular_velocity = -2
  (default) -> FollowTrack
  FollowTrack -> TurnLeft [order 1] : [IR2 == 0]
  TurnRight -> FollowTrack : [IR3 == 1 && IR2 == 1]
  TurnLeft -> FollowTrack : [IR3 == 1 && IR2 == 1]
  FollowTrack -> TurnRight [order 2] : [IR3 == 0]
  data: velocity output; angular_velocity output; IR2 input; IR3 input

== stateflow chart Milestone3_Code_JanasWork/Object Detection/Measure Objects ==
  state sendTrigger
    %output trigger High to start measurement
    entry: trigger = 1;
    exit: trigger = 0;
    start = elapsed(sec);
  state measureEcho
    %calculate time elapsed between trigger sent
    %and echo received
    if echo == 1
    finish = elapsed(sec);
    timeElapsed = finish + start;
    end
  state calculateAndCompareDistance
    %calculate distance from timeElapsed
    entry: distance = timeElapsed*0.344/2;
    during:
    %pick shortest distance
    if distance < smallestDistance || smallestDistance == -1
    smallestDistance = distance;
    objectCounter = objectCounter + 1;
    end
    smallestDistance = distance;
    MeasurementComplete =1;
  state ChillingState
    %waiting for measure command
    %from line sensing
    entry:
    MeasurementComplete =0;
    timeElapsed = 0;
  state Wait
    %wait for measure command
    %to end
  (junction 98) -> sendTrigger : [detectObject ==1]
  ChillingState -> (junction 98)
  sendTrigger -> measureEcho : after(10, usec)
  (default) -> ChillingState
  measureEcho -> (junction 100) : [timeElapsed > 0]
  (junction 100) -> calculateAndCompareDistance
  Wait -> ChillingState : after(3,sec) %[detectObject==0]
  calculateAndCompareDistance -> Wait : [MeasurementComplete ==1]
  data: detectObject input; smallestDistance output =-1; objectCounter output =0; trigger output =0; timeElapsed local =0; start local; finish local; distance local size=1 =0; echo input; MeasurementComplete output =0

== stateflow chart Milestone3_Code_JanasWork/Motion Control1/Intersection Navigation ==
  note: Basic Description
      | Default: Curve Navigation controls the velocity and angular velocity
      |
      | When infrared sensor 1 or 4 (IR1 and IR4) detect a black line, this Intersection Navigation subsystem takes control and calls the leftTurn or rightTurn procedure respectively.
      | Intersection procedure (same for both leftTurn or rightTurn):
      | 	Increment branchCounter to keep track of the number of branches.
      | 	Move forward a small distance to align with the turn.
      | 	Rotate in the correct direction until the middle two sensors detect a line again.
      | 	Pass control to Curve Navigation to navigate the offshoot.
      | 	If the offshoot comes to an end (all sensors detect white), rotate 180 degrees and navigate back to the main path.
      | 	If the offshoot ends in a detect line (all sensors detect black), stop, send a signal to the Object Detection subsystem to measure for an object, rotate 180 degrees and navigate back to the main path.
      | 		Add branch number from branchCounter to objectMap to indicate this branch has an object.
      | 	Pass control to Curve Navigation to navigate the offshoot returning to the main path.
      | 	When the peripheral sensors detect a black line again (meaning the robot has returned to the intersection with the main branch), control is passed to Intersection Navigation.
      | 	Move forward a small distance to align with the turn.
      | 	Rotate in the correct direction until the middle two sensors detect a line again.
      | 	Pass control back to Curve Navigation to continue traversing the main path.
      |
      | If all sensors detect black whilst the robot is on the main path, the endOfMaze procedure is called.
      | endOfMaze procedure:
      | 	Stop
      | 	Use objectMap to determine how many objects were discovered.
      | 	Find the branch number of the object with the smallest distance, saved to branchWithObject.
      | 		objectCounter provides number of object with smallest distance measured.
      | 		Obtain the n'th number in objectMap to determine the branch number containing said object (where n = objectCounter)
      | 	Invert branchWithObject such that it provides the number of the branch starting from the end of the maze.
      | 	Set renavigating to HIGH.
      |
      | Renavigating Procedure:
      | 	Rotate 180 degrees to re-traverse the maze.
      | 	set branchCounter to 0.
      | 	Pass control to Curve Navigation to renavigate maze.
      | 	If intersection is detected, increment branchCounter.
      | 	If branchCounter is equal to branchWithObject at an intersection, turn into that offshoot.
      | 	Pass control to Curve Navigation to navigate offshoot.
      | 	If all sensors detect black at the "detect object line", come to a stop.
  state endOfMaze
    %procedure to locate position of closest object once maze is completed
    entry: navigatingIntersection = 1;
    velocity = 0;
    angular_velocity = 0;
    num = objectMap;
    while num > 0
    len = len + 1;
    num = fix(num/10);
    end
    branchWithObject = mod(fix(objectMap/10^(len - objectCounter)), 10);
    branchWithObject = branchCounter - branchWithObject + 1;
    exit:
    renavigating = 1;
  state fullRotation
    %rotate 180 degrees to renavigate maze
    entry: phi0 = phi;
    during:
    velocity = 0;
    angular_velocity = -4;
  state mainPath
    %Control given to Curve Navigation Subsystem
    entry: navigatingIntersection = 0;
  state rightTurn
    %procedure for navigating an offshoot to the right of the main path
    state returnToMain
      entry: navigatingIntersection = 0;
    state rightToMain
      %turn right back onto the main path
      entry: phi0 = phi;
      during:
      velocity = 0.1;
      angular_velocity = -4;
    state alignWithTurn
      entry: distance0 = distance;
      branchCounter = branchCounter +1;
      exit: navigatingIntersection = 1;
    state alignWithMain
      entry: distance0 = distance;
      exit: navigatingIntersection = 1;
    state rotate
      %turn right
      entry:
      phi0 = phi;
      during:
      velocity = 0.1;
      angular_velocity = -4;
    state navigateOffshoot
      entry: navigatingIntersection = 0;
      exit: navigatingIntersection = 1;
    state stopAndMeasure
      entry:
      velocity = 0;
      angular_velocity = 0;
      collectMeasurement = 1;
      exit:
      collectMeasurement = 0;
    state fullRotation
      %rotate 180 degrees
      entry: phi0 = phi;
      during:
      velocity = 0;
      angular_velocity = -4;
    state finalStop
      velocity = 0;
      angular_velocity = 0;
    (default) -> rightTurn.alignWithTurn
    rightTurn.alignWithMain -> rightToMain : [abs(distance - distance0) > 0.01]
    rightTurn.returnToMain -> rightTurn.alignWithMain : [IR4 == 0]
    rightTurn.alignWithTurn -> rightTurn.rotate : [abs(distance - distance0) > 0.005]
    rightTurn.fullRotation -> rightTurn.returnToMain : [abs(phi - phi0) > 2.793 && abs(phi - phi0) < 3.491 && IR2 == 0 && IR3 == 0]
    rightTurn.rotate -> rightTurn.navigateOffshoot : [((abs(phi - phi0) > 0.3491 && abs(phi - phi0) < 2.967) || (abs(phi - phi0) > 3.316 && abs(phi - phi0) < 5.934)) && IR2 == 0 && IR3 == 0]
    rightTurn.navigateOffshoot -> (junction 254) [order 1]
    rightTurn.navigateOffshoot -> (junction 194) [order 3] : [IR1 == 1 && IR2 == 1 && IR3 == 1 && IR4 == 1]
    (junction 254) -> (junction 256) : [IR1 + IR2 + IR3 + IR4 == 0 && renavigating == 1]
    (junction 194) -> rightTurn.fullRotation
    rightTurn.navigateOffshoot -> rightTurn.stopAndMeasure [order 2] : [IR1 == 0 && IR2 == 0 && IR3 == 0 && IR4 ==0]{objectMap = objectMap*10 + branchCounter;} %detect or stop line
    rightTurn.stopAndMeasure -> rightTurn.fullRotation : [measurementComplete == 1]
    (junction 256) -> rightTurn.finalStop
  state leftTurn
    %procedure for navigating an offshoot to the right of the main path
    state leftToMain
      %turn left back onto the main path
      entry: phi0 = phi;
      during:
      velocity = 0.1;
      angular_velocity = 4;
    state returnToMain
      entry: navigatingIntersection = 0;
    state alignWithTurn
      entry: distance0 = distance;
      branchCounter = branchCounter +1;
      exit: navigatingIntersection = 1;
    state alignWithMain
      entry: distance0 = distance;
      exit: navigatingIntersection = 1;
    state rotate
      %turn left
      entry:
      phi0 = phi;
      during:
      velocity = 0.1;
      angular_velocity = 4;
    state navigateOffshoot
      entry: navigatingIntersection = 0;
      exit: navigatingIntersection = 1;
    state stopAndMeasure
      entry:
      velocity = 0;
      angular_velocity = 0;
      collectMeasurement = 1;
      exit:
      collectMeasurement = 0;
    state fullRotation
      %rotate 180 degrees
      entry: phi0 = phi;
      during:
      velocity = 0;
      angular_velocity = -4;
    state finalStop
      velocity = 0;
      angular_velocity = 0;
    (default) -> leftTurn.alignWithTurn
    leftTurn.alignWithMain -> leftToMain : [abs(distance - distance0) > 0.01]
    leftTurn.returnToMain -> leftTurn.alignWithMain : [IR1 == 0]
    leftTurn.alignWithTurn -> leftTurn.rotate : [abs(distance - distance0) > 0.005]
    leftTurn.fullRotation -> leftTurn.returnToMain : [abs(phi - phi0) > 2.793 && abs(phi - phi0) < 3.491 && IR2 == 0 && IR3 == 0]
    leftTurn.rotate -> leftTurn.navigateOffshoot : [((abs(phi - phi0) > 0.3491 && abs(phi - phi0) < 2.967) || (abs(phi - phi0) > 3.316 && abs(phi - phi0) < 5.934)) && IR2 == 0 && IR3 == 0]
    leftTurn.navigateOffshoot -> (junction 216) [order 3] : [IR1 == 1 && IR2 == 1 && IR3 == 1 && IR4 == 1]
    leftTurn.navigateOffshoot -> (junction 263) [order 1]
    (junction 216) -> leftTurn.fullRotation
    (junction 263) -> (junction 264) : [IR1 + IR2 + IR3 + IR4 == 0 && renavigating == 1]
    leftTurn.navigateOffshoot -> leftTurn.stopAndMeasure [order 2] : [IR1 == 0 && IR2 == 0 && IR3 == 0 && IR4 ==0]{objectMap = objectMap*10 + branchCounter;} %detect or stop line
    leftTurn.stopAndMeasure -> leftTurn.fullRotation : [measurementComplete == 1]
    (junction 264) -> leftTurn.finalStop
  state renavigatingCounter
    entry:
    branchCounter = branchCounter + 1;
  endOfMaze -> fullRotation : {branchCounter = 0;}
  fullRotation -> mainPath : [abs(phi - phi0) > 2.793 && abs(phi - phi0) < 3.491 && IR2 == 0 && IR3 == 0]
  mainPath -> endOfMaze [order 1] : [IR1 + IR2 + IR3 + IR4 == 0]
  (default) -> mainPath
  (junction 225) -> mainPath
  (junction 197) -> mainPath
  leftToMain -> (junction 225) : [((abs(phi - phi0) > 0.3491 && abs(phi - phi0) < 2.967) || (abs(phi - phi0) > 3.316 && abs(phi - phi0) < 5.934)) && IR2 == 0 && IR3 == 0]
  rightToMain -> (junction 197) : [((abs(phi - phi0) > 0.3491 && abs(phi - phi0) < 2.967) || (abs(phi - phi0) > 3.316 && abs(phi - phi0) < 5.934)) && IR2 == 0 && IR3 == 0]
  mainPath -> (junction 223) [order 3] : [IR1 == 0 && IR2 == 0 && IR3 == 0 && IR4 == 1 && ((renavigating == 0) || (renavigating == 1 && branchCounter == branchWithObject) )]
  renavigatingCounter -> mainPath [order 3] : [IR1 == 1 && IR4 == 1]
  mainPath -> renavigatingCounter [order 4] : [(IR1 == 0 || IR4 == 0) && renavigating == 1]
  mainPath -> (junction 199) [order 2] : [IR1 == 1 && IR2 == 0 && IR3 == 0 && IR4 == 0 && ((renavigating == 0) || (renavigating == 1 && branchCounter == branchWithObject) )]
  (junction 223) -> leftTurn
  (junction 199) -> rightTurn
  renavigatingCounter -> rightTurn.rotate [order 1] : [IR4 == 0 && branchCounter == branchWithObject]{navigatingIntersection = 1;}
  renavigatingCounter -> leftTurn.rotate [order 2] : [IR1 == 0 && branchCounter == branchWithObject]{navigatingIntersection = 1;}
  data: len local =0; num local =0; velocity output; angular_velocity output; IR1 input; IR2 input; IR3 input; IR4 input; navigatingIntersection output; collectMeasurement output; phi input; phi0 local; distance input; distance0 local =0; objectCounter input; objectMap output =0; branchCounter local =0; branchWithObject local =0; renavigating local =0; measurementComplete input
